simulink model "liftsubsystem"  (R2025b)
settings: Solver=daessc  StartTime=0.0  StopTime=15  FixedStep=1e-3  RelTol=1e-3
values from neighbouring files (symbols this model uses):
  b0 = 1.0    (= 1)    [get_arm_model_with_disturbance.m]    (also in robotParams.m = 3.125)
  beta1 = 3 * omega_o    (= 120)    [robotParams.m]
  beta2 = 3 * omega_o^2    (= 4800)    [robotParams.m]
  beta3 = omega_o^3    (= 64000)    [robotParams.m]
  g = 9.81    [get_arm_model.m]    (also in robotParams.m)
  g_fork = 2*pi*50    (= 314.159265359)    [robotParams.m]
  g_lift = 2*pi*50    (= 314.159265359)    [robotParams.m]
  Kd_fork = 5    [robotParams.m]
  Kd_lift = 5    [robotParams.m]
  Kp_fork = 20    [robotParams.m]
  Kp_lift = 20    [robotParams.m]
  lx = 0.3    [robotParams.m]
  ly = 0.8    [robotParams.m]
  lz = 1    [robotParams.m]
  m = 1    [robotParams.m]
  M = reshape([mt1,mt2,mt3],4,4)    [mass_matrix.m]    (also in robotParams.m = 16)
  m_w = 1    [robotParams.m]
  N = 20    [ocp_arm.m]    (also in ocp_arm_disturbances.m; ocp_lift.m)
  T_control = 1e-3    (= 0.001)    [robotParams.m]
undefined symbols (not defined in the file or in its folder): dspblkCoreblockFVToolHelper, gcbh, K_fd, K_fp, M_n44, Mn_33, Mn_44, X, Y, Z
libraries: sm_lib x257, nesl_utility x58, sharedTrackingLibrary x6, slpidlib x4, simulink x4, robotcorelib x1
(part 8 of 8)

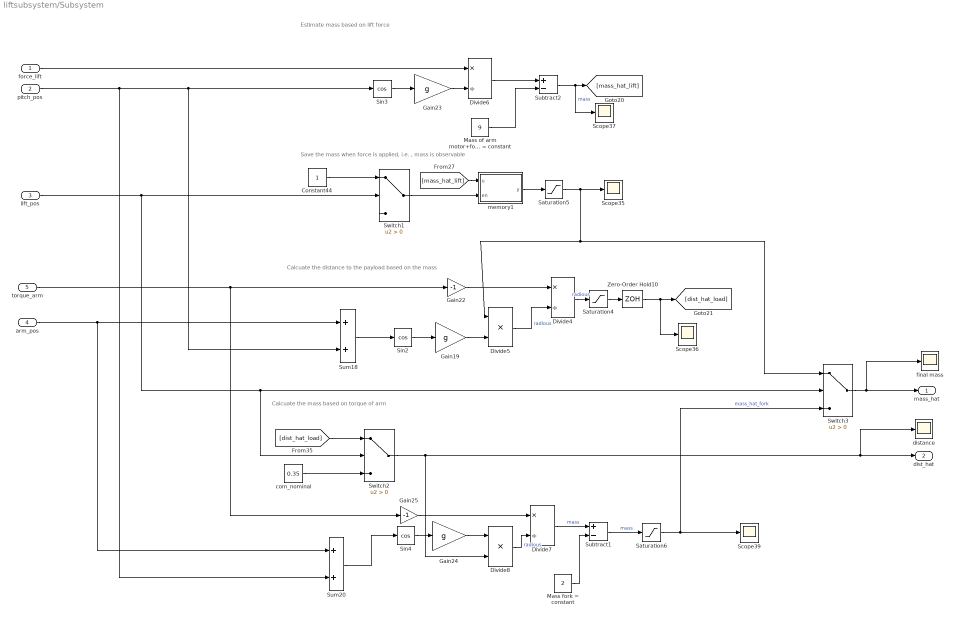
== system liftsubsystem/Subsystem ==
  note: Estimate mass based on lift force
  note: Save the mass when force is applied, i.e. , mass is observable
  note: Calcuate the distance to the payload based on the mass
  note: Calcuate the mass based on torque of arm
  force_lift : Inport
  pitch_pos : Inport  Port=2
  lift_pos : Inport  Port=3
  arm_pos : Inport  Port=4
  torque_arm : Inport  Port=5
  Constant44 : Constant
  Divide4 : Product  Inputs=*/
  Divide5 : Product  Inputs=**
  Divide6 : Product  Inputs=*/
  Divide7 : Product  Inputs=*/
  Divide8 : Product  Inputs=**
  Gain19 : Gain  Gain=g
  Gain22 : Gain  Gain=-1
  Gain23 : Gain  Gain=g
  Gain24 : Gain  Gain=g
  Gain25 : Gain  Gain=-1
  Mass fork = constant : Constant  Value=2
  Mass of arm motor+fork = constant : Constant  Value=9
  Saturation4 : Saturate  UpperLimit=0.6  LowerLimit=0.1
  Saturation5 : Saturate  UpperLimit=20  LowerLimit=0
  Saturation6 : Saturate  UpperLimit=20  LowerLimit=0
  Scope{35..37,39} (4 alike) : Scope
      Scope35 settings: ActiveDisplayYMinimum=-1.2708762754885328  ActiveDisplayYMaximum=14.804410070172921  DataLoggingVariableName=ScopeData41
      Scope36 settings: ActiveDisplayYMinimum=-0.0615737983063222  ActiveDisplayYMaximum=3.0231286948708305  DataLoggingVariableName=ScopeData42
      Scope37 settings: ActiveDisplayYMinimum=-4.9295636501203735  ActiveDisplayYMaximum=16.727099942606021  DataLoggingVariableName=ScopeData43
      Scope39 settings: ActiveDisplayYMinimum=-0.718038981848304  ActiveDisplayYMaximum=31.278716537533729  DataLoggingVariableName=ScopeData45
  Sin2 : Trigonometry  Operator=cos
  Sin3 : Trigonometry  Operator=cos
  Sin4 : Trigonometry  Operator=cos
  Subtract1 : Sum  Inputs=+-
  Subtract2 : Sum  Inputs=+-
  Sum18 : Sum
  Sum20 : Sum
  Switch1 : Switch  Criteria=u2 > Threshold  SaturateOnIntegerOverflow=off  InputSameDT=off
  Switch2 : Switch  Criteria=u2 > Threshold  SaturateOnIntegerOverflow=off  InputSameDT=off
  Switch3 : Switch  Criteria=u2 > Threshold  SaturateOnIntegerOverflow=off  InputSameDT=off
  Zero-Order Hold10 : ZeroOrderHold  SampleTime=-1
  com_nominal : Constant  Value=0.35
  distance : Scope
      settings: ActiveDisplayYMinimum=0.32424406541533968  ActiveDisplayYMaximum=0.38026879483052378  DataLoggingVariableName=ScopeData47
  final mass : Scope
      settings: ActiveDisplayYMinimum=1.0929972674298374  ActiveDisplayYMaximum=6.2989898621866436  DataLoggingVariableName=ScopeData46
  memory1 : MATLAB Function  TreatAsAtomicUnit=on
  mass_hat : Outport
  dist_hat : Outport  Port=2
  wires:
  Constant44/1 -> Switch1/1
  memory1/1(y) -> Saturation5/1
  pitch_pos/1 -> Sum20/2, Sin3/1, Sum18/2
  lift_pos/1 -> Switch1/2, Switch2/2, Switch3/2
  com_nominal/1 -> Switch2/3
  Divide5/1 -> Divide4/2  "radious"
  force_lift/1 -> Divide6/1
  [mass_hat_lift] -> memory1/1(u)
  Switch1/1 -> memory1/2(en)
  Zero-Order Hold10/1 -> [dist_hat_load], Scope36/1
  [dist_hat_load] -> Switch2/1
  Sin4/1 -> Gain24/1
  Switch2/1 -> dist_hat/1, distance/1, Divide8/2
  Sin3/1 -> Gain23/1
  arm_pos/1 -> Sum20/1, Sum18/1
  Saturation5/1 -> Divide5/1, Switch3/1, Scope35/1
  Saturation4/1 -> Zero-Order Hold10/1
  Divide4/1 -> Saturation4/1  "radious"
  torque_arm/1 -> Gain22/1, Gain25/1
  Sum20/1 -> Sin4/1
  Saturation6/1 -> Switch3/3, Scope39/1  "mass_hat_fork"
  Sin2/1 -> Gain19/1
  Switch3/1 -> mass_hat/1, final mass/1
  Gain25/1 -> Divide7/1
  Divide6/1 -> Subtract2/1
  Gain22/1 -> Divide4/1
  Divide7/1 -> Subtract1/1  "mass"
  Gain24/1 -> Divide8/1
  Divide8/1 -> Divide7/2  "radious"
  Mass of arm motor+fork = constant/1 -> Subtract2/2
  Sum18/1 -> Sin2/1
  Gain19/1 -> Divide5/2
  Subtract2/1 -> Scope37/1, [mass_hat_lift]  "mass"
  Gain23/1 -> Divide6/2
  Mass fork = constant/1 -> Subtract1/2
  Subtract1/1 -> Saturation6/1  "mass"

== system liftsubsystem/Calculations/myDerivative1 ==
  In1 : Inport
  Delay3 : Delay  DelayLength=1  InputProcessing=Columns as channels (frame based)
  Gain23 : Gain  Gain=1/T_control
  Subtract2 : Sum  Inputs=+-
  Out1 : Outport
  wires:
  Gain23/1 -> Out1/1
  Subtract2/1 -> Gain23/1
  Delay3/1 -> Subtract2/2
  In1/1 -> Subtract2/1, Delay3/1

== system liftsubsystem/Calculations/myDerivative2 ==
  In1 : Inport
  Delay3 : Delay  DelayLength=1  InputProcessing=Columns as channels (frame based)
  Gain23 : Gain  Gain=1/T_control
  Subtract2 : Sum  Inputs=+-
  Out1 : Outport
  wires:
  Gain23/1 -> Out1/1
  Subtract2/1 -> Gain23/1
  Delay3/1 -> Subtract2/2
  In1/1 -> Subtract2/1, Delay3/1

== system liftsubsystem/Calculations/myDerivative3 ==
  In1 : Inport
  Delay3 : Delay  DelayLength=1  InputProcessing=Columns as channels (frame based)
  Gain23 : Gain  Gain=1/T_control
  Subtract2 : Sum  Inputs=+-
  Out1 : Outport
  wires:
  In1/1 -> Delay3/1, Subtract2/1
  Delay3/1 -> Subtract2/2
  Subtract2/1 -> Gain23/1
  Gain23/1 -> Out1/1

== system liftsubsystem/Calculations/myDerivative4 ==
  In1 : Inport
  Delay3 : Delay  DelayLength=1  InputProcessing=Columns as channels (frame based)
  Gain23 : Gain  Gain=1/T_control
  Subtract2 : Sum  Inputs=+-
  Out1 : Outport
  wires:
  Gain23/1 -> Out1/1
  Subtract2/1 -> Gain23/1
  Delay3/1 -> Subtract2/2
  In1/1 -> Subtract2/1, Delay3/1

== system liftsubsystem/Calculations/myDerivative5 ==
  In1 : Inport
  Delay3 : Delay  DelayLength=1  InputProcessing=Columns as channels (frame based)
  Gain23 : Gain  Gain=1/T_control
  Subtract2 : Sum  Inputs=+-
  Out1 : Outport
  wires:
  In1/1 -> Delay3/1, Subtract2/1
  Delay3/1 -> Subtract2/2
  Subtract2/1 -> Gain23/1
  Gain23/1 -> Out1/1

== matlab function liftsubsystem/MATLAB Function ==
  data: mass input; cog_new output; distance input; height input
function cog_new = cog_new(mass, distance, height)
    % Fixed previous mass and center of gravity
    mass_old = 28;
    cog_old = [-0.0232, 0, 0.857];

    % Offset introduced by the new mass
    offset = cog_old + [distance, 0, height];

    % New center of gravity (mass-weighted average)
    cog_new = (mass_old * cog_old + mass * offset) / (mass + mass_old);
end

== matlab function liftsubsystem/Subsystem/memory1 ==
  settings: updateMethod=DISCRETE
  data: u input; y output; en input
function y = fcn(u,en)
persistent mem
if isempty(mem)
    mem = 0; % valor inicial
end
if en
    mem = u;
end
y = mem;
end
